simulink model "propultion"  (R2022a)
settings: Solver=VariableStepAuto  StartTime=0.0  StopTime=3600  RelTol=1e-3
undefined symbols (not defined in the file): h, km, m, s
libraries: simulink x5, simulink_extras x1, aerolibconvert2 x1
settings Model: Creator=User  LastModifiedBy=User

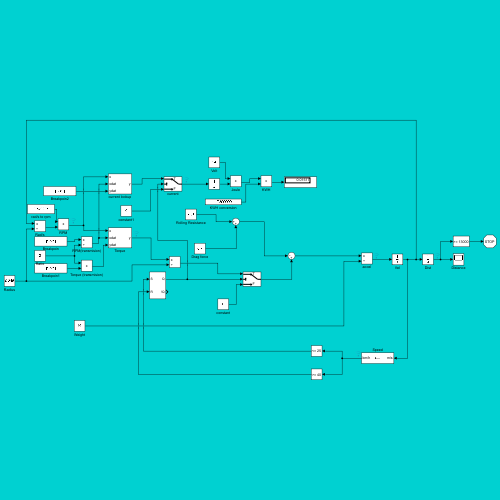
[thumbnail: Simulink's stored preview of the top-level diagram]
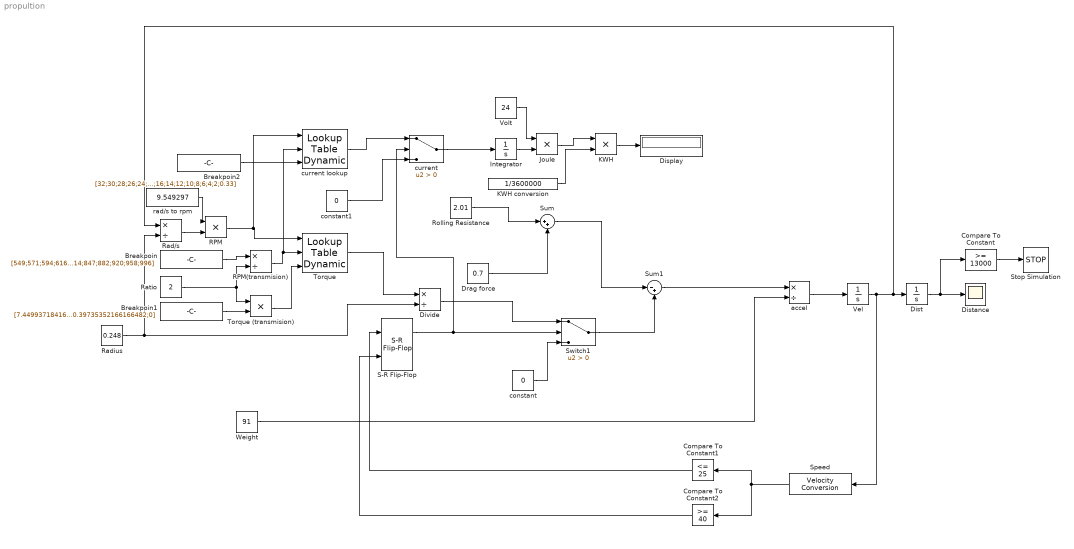
== system propultion ==
  Breakpoin : Constant  Value=[549;571;594;616;639;660;682;705;730;756;784;814;847;882;920;958;996]
  Breakpoin1 : Constant  Value=[7.4499371841666315;7.1109826961666336;6.7674381994749684;6.4059573611266361;6.0254809483466385;5.6153460178666403;5.1735753351733091;4.6820913275733114;4.1476730848266472;3.613254842079983;3.0641485715199859;2.5082632111999881;1.9467286094133243;1.4179596081333268;0.88940245340832913;0.39735352166166482;0]
  Breakpoin2 : Constant  Value=[32;30;28;26;24;22;20;18;16;14;12;10;8;6;4;2;0.33]
  Compare To Constant : simulink/Logic and Bit Operations/Compare To Constant  relop=>=  const=13000  OutDataTypeStr=boolean
  Compare To Constant1 : simulink/Logic and Bit Operations/Compare To Constant  relop=<=  const=25  OutDataTypeStr=boolean
  Compare To Constant2 : simulink/Logic and Bit Operations/Compare To Constant  relop=>=  const=40  OutDataTypeStr=boolean
  Display : Display
  Dist : Integrator
  Distance : Scope
  Divide : Product  Inputs=*/
  Drag force : Constant  Value=0.7
  Integrator : Integrator
  Joule : Product
  KWH : Product
  KWH conversion : Constant  Value=1/3600000
  RPM : Product
  RPM(transmision) : Product  Inputs=*/
  Rad/s : Product  Inputs=*/
  Radius : Constant  Value=0.248
  Ratio : Constant  Value=2
  Rolling Resistance : Constant  Value=2.01
  S-R Flip-Flop : simulink_extras/Flip Flops/S-R Flip-Flop  initial_condition=0
  Speed : aerolibconvert2/Velocity Conversion  IU=m/s  OU=km/h
  Stop Simulation : Stop
  Sum : Sum  Inputs=|++
  Sum1 : Sum  Inputs=|-+
  Switch1 : Switch  Criteria=u2 > Threshold  SaturateOnIntegerOverflow=off  InputSameDT=off
  Torque : simulink/Lookup Tables/Lookup Table Dynamic  LookUpMeth=Interpolation-Extrapolation  OutDataType=fixdt('double')  OutScaling=2^-10  OutputDataTypeScalingMode=Specify via dialog  OutDataTypeStr=double  DoSatur=off
  Torque (transmision) : Product
  Vel : Integrator
  Volt : Constant  Value=24
  Weight : Constant  Value=91
  accel : Product  Inputs=*/
  constant : Constant  Value=0
  constant1 : Constant  Value=0
  current : Switch  Criteria=u2 > Threshold  SaturateOnIntegerOverflow=off  InputSameDT=off
  current lookup : simulink/Lookup Tables/Lookup Table Dynamic  LookUpMeth=Interpolation-Use End Values  OutDataType=fixdt('double')  OutScaling=2^-10  OutputDataTypeScalingMode=Specify via dialog  OutDataTypeStr=double  DoSatur=off
  rad/s to rpm : Constant  Value=9.549297
  wires:
  Drag force/1 -> Sum/2
  Radius/1 -> Divide/2, Rad/s/2
  Weight/1 -> accel/2
  accel/1 -> Vel/1
  Vel/1 -> Speed/1, Rad/s/1, Dist/1
  Dist/1 -> Compare To Constant/1, Distance/1
  Compare To Constant/1 -> Stop Simulation/1
  Sum/1 -> Sum1/1
  Sum1/1 -> accel/1
  S-R Flip-Flop/1 -> current/2, Switch1/2
  Divide/1 -> Switch1/1
  constant/1 -> Switch1/3
  Switch1/1 -> Sum1/2
  Compare To Constant1/1 -> S-R Flip-Flop/1
  Compare To Constant2/1 -> S-R Flip-Flop/2
  Speed/1 -> Compare To Constant1/1, Compare To Constant2/1
  Rolling Resistance/1 -> Sum/1
  Torque/1 -> Divide/1
  RPM(transmision)/1 -> current lookup/2, Torque/2
  Breakpoin/1 -> RPM(transmision)/1
  Ratio/1 -> RPM(transmision)/2, Torque (transmision)/1
  Breakpoin1/1 -> Torque (transmision)/2
  Torque (transmision)/1 -> Torque/3
  Breakpoin2/1 -> current lookup/3
  Integrator/1 -> Joule/2
  Volt/1 -> Joule/1
  KWH conversion/1 -> KWH/2
  Joule/1 -> KWH/1
  KWH/1 -> Display/1
  Rad/s/1 -> RPM/2
  RPM/1 -> current lookup/1, Torque/1
  rad/s to rpm/1 -> RPM/1
  current lookup/1 -> current/1
  constant1/1 -> current/3
  current/1 -> Integrator/1
